simulink model "Modele_LQR_6DOF"  (R2024b)
settings: Solver=VariableStepAuto  StartTime=0.0  StopTime=50  FixedStep=0.0001  RelTol=1e-3
InitFcn:
  |     du0 = 0;
  |     du1 = 0;
  |     du2 = 0;
  |     du3 = 0;
  |     du4 = 0;
  |     du5 = 0;
  |     du6 = 0;
  |     du7 = 0;
values from neighbouring files (symbols this model uses):
  A_num = [0 0 0 0 0 0 0 0 0 0 0 0 ... (144 elements, 12x12)]    [Matrice_A_lineaire.mat]    (also in calcul_matrice_A_lineaire.m = double(A_num); resultats_stabilite.mat; testFinale.m = A_fcn(0, 0, 0, val_rll, val_ptc, val_yw, val_u, val_v, val_w; test_calcalV2.m = double(A_num))
  B = df_dcontrol    [Generate_PyMatrix.m]    (also in Parameters.m = -234.459; instabiliter_graphique.m = out.B_s.signals.values)
  Fx1 = -0.7071*force    (= -14.142)    [Parameters.m]
  Fx2 = -0.7071*force    (= -14.142)    [Parameters.m]
  Fx3 = 0    [Parameters.m]
  Fx4 = 0    [Parameters.m]
  Fx5 = 0    [Parameters.m]
  Fx6 = 0    [Parameters.m]
  Fx7 = 0.7071*force    (= 14.142)    [Parameters.m]
  Fx8 = 0.7071*force    (= 14.142)    [Parameters.m]
  Fy1 = 0.7071*force    (= 14.142)    [Parameters.m]
  Fy2 = -0.7071*force    (= -14.142)    [Parameters.m]
  Fy3 = 0    [Parameters.m]
  Fy4 = 0    [Parameters.m]
  Fy5 = 0    [Parameters.m]
  Fy6 = 0    [Parameters.m]
  Fy7 = 0.7071*force    (= 14.142)    [Parameters.m]
  Fy8 = -0.7071*force    (= -14.142)    [Parameters.m]
  Fz1 = 0    [Parameters.m]
  Fz2 = 0    [Parameters.m]
  Fz3 = -1*force    (= -20)    [Parameters.m]
  Fz4 = -1*force    (= -20)    [Parameters.m]
  Fz5 = -1*force    (= -20)    [Parameters.m]
  Fz6 = -1*force    (= -20)    [Parameters.m]
  Fz7 = 0    [Parameters.m]
  Fz8 = 0    [Parameters.m]
  I_x = 0.578    [Parameters.m]
  I_y = 0.645    [Parameters.m]
  I_z = 0.9366    [Parameters.m]
  lx1 = I_un_moteur(1)    [Calcul_Inertie_Nouveau.m]    (also in Parameters.m = 0.0194)
  lx2 = I_un_moteur(1)    [Calcul_Inertie_Nouveau.m]    (also in Parameters.m = 0.0194)
  lx3 = I_un_moteur(1)    [Calcul_Inertie_Nouveau.m]    (also in Parameters.m = -0.0317)
  lx4 = I_un_moteur(1)    [Calcul_Inertie_Nouveau.m]    (also in Parameters.m = -0.0317)
  lx5 = I_un_moteur(1)    [Calcul_Inertie_Nouveau.m]    (also in Parameters.m = 0.0317)
  lx6 = I_un_moteur(1)    [Calcul_Inertie_Nouveau.m]    (also in Parameters.m = 0.0317)
  lx7 = I_un_moteur(1)    [Calcul_Inertie_Nouveau.m]    (also in Parameters.m = -0.0194)
  lx8 = I_un_moteur(1)    [Calcul_Inertie_Nouveau.m]    (also in Parameters.m = -0.0194)
  ly1 = %.4f    [Calcul_Inertie_Nouveau.m]    (also in Parameters.m = 0.0381)
  ly2 = %.4f    [Calcul_Inertie_Nouveau.m]    (also in Parameters.m = -0.0381)
  ly3 = %.4f    [Calcul_Inertie_Nouveau.m]    (also in Parameters.m = 0.0049)
  ly4 = %.4f    [Calcul_Inertie_Nouveau.m]    (also in Parameters.m = -0.0049)
  ly5 = %.4f    [Calcul_Inertie_Nouveau.m]    (also in Parameters.m = 0.0049)
  ly6 = %.4f    [Calcul_Inertie_Nouveau.m]    (also in Parameters.m = -0.0049)
  ly7 = %.4f    [Calcul_Inertie_Nouveau.m]    (also in Parameters.m = 0.0381)
  ly8 = %.4f    [Calcul_Inertie_Nouveau.m]    (also in Parameters.m = -0.0381)
  lz1 = %.4f;\n', lx1, ly1, lz1)    [Calcul_Inertie_Nouveau.m]    (also in Parameters.m = 0.0575)
  lz2 = %.4f;\n', lx2, ly2, lz2)    [Calcul_Inertie_Nouveau.m]    (also in Parameters.m = 0.0575)
  lz3 = %.4f;\n', lx3, ly3, lz3)    [Calcul_Inertie_Nouveau.m]    (also in Parameters.m = 0.0366)
  lz4 = %.4f;\n', lx4, ly4, lz4)    [Calcul_Inertie_Nouveau.m]    (also in Parameters.m = 0.0366)
  lz5 = %.4f;\n', lx5, ly5, lz5)    [Calcul_Inertie_Nouveau.m]    (also in Parameters.m = 0.0366)
  lz6 = %.4f;\n', lx6, ly6, lz6)    [Calcul_Inertie_Nouveau.m]    (also in Parameters.m = 0.0366)
  lz7 = %.4f;\n', lx7, ly7, lz7)    [Calcul_Inertie_Nouveau.m]    (also in Parameters.m = 0.0575)
  lz8 = %.4f;\n', lx8, ly8, lz8)    [Calcul_Inertie_Nouveau.m]    (also in Parameters.m = 0.0575)
  m = 23.9    [Parameters.m]
  Q_envoyer = Q_final(:,:,1)    [Parameters.m]
  W = mass*gravity    (= 234.459)    [Generate_PyMatrix.m]    (also in Parameters.m; calcul_damping.m)
  x_rb = 0    [Parameters.m]
  x_rg = 0    [Parameters.m]
  y_rb = 0    [Parameters.m]
  y_rg = 0    [Parameters.m]
  z_rb = 0    [Parameters.m]
  z_rg = 0    [Parameters.m]
undefined symbols (not defined in the file or in its folder): sigbuilder_block
libraries: simulink x12, sharedtransform x1, dspinverses x1, SignalEditorBlockLib x1
(part 2 of 4)

== matlab function Modele_LQR_6DOF/ROV model/ROV model/Kinetics1 ==
  data: u input size=1; u_dot output; v input size=1; w input size=1; p input size=1; q input size=1; r input size=1; phi input; theta input; psi input; tau input; v_dot output; w_dot output; p_dot output; q_dot output; r_dot output; u_dot_temp input; v_dot_temp input; w_dot_temp input; p_dot_temp input; q_dot_temp input; r_dot_temp input; disturbance input; EstimatedParams input; B parameter; Fx1 input; Fx2 input; Fx3 input; Fx4 input; Fx5 input; Fx6 input; Fx7 input; Fx8 input; Fy1 input; Fy2 input; Fy3 input; Fy4 input; Fy5 input; Fy6 input; Fy7 input; Fy8 input; Fz1 input; Fz2 input; Fz3 input; Fz4 input; Fz5 input; Fz6 input; Fz7 input; Fz8 input; I_x input; I_y input; I_z input; lx1 input; lx2 input; lx3 input; lx4 input; lx5 input; lx6 input; lx7 input; lx8 input; ly1 input; ly2 input; ly3 input; ly4 input; ly5 input; ly6 input; ly7 input; ly8 input; lz1 input; lz2 input; lz3 input; lz4 input; lz5 input; lz6 input; lz7 input; lz8 input; m parameter; W parameter; x_rb parameter; x_rg parameter; y_rb parameter; y_rg parameter; z_rb parameter; z_rg parameter
function [u_dot,v_dot,w_dot,p_dot,q_dot,r_dot] = Kinetics1(u,v,w,p,q,r,phi,theta,psi,tau,u_dot_temp,v_dot_temp,w_dot_temp,p_dot_temp,q_dot_temp,r_dot_temp, disturbance,EstimatedParams, B, Fx1, Fx2, Fx3, Fx4, Fx5, Fx6, Fx7, Fx8, Fy1, Fy2, Fy3, Fy4, Fy5, Fy6, Fy7, Fy8, Fz1, Fz2, Fz3, Fz4, Fz5, Fz6, Fz7, Fz8, I_x, I_y, I_z, lx1, lx2, lx3, lx4, lx5, lx6, lx7, lx8, ly1, ly2, ly3, ly4, ly5, ly6, ly7, ly8, lz1, lz2, lz3, lz4, lz5, lz6, lz7, lz8, m, W, x_rb, x_rg, y_rb, y_rg, z_rb, z_rg)
% LIVRE HMCH PAGE 58
%extract forces from thrusters
f1=tau(1);
f2=tau(2);
f3=tau(3);
f4=tau(4);
f5=tau(5);
f6=tau(6);
f7=tau(7);
f8=tau(8);
x_rb = 0; x_rg = 0; y_rb = 0; y_rg = 0; z_rb = -0.05; z_rg = 0;
  displaced_water_volume = 0.024; % 0.03
  water_density = 1000.0;
  radius = 0.26;
  m = 23.9;
  g = 9.81;
  W = m * g;
  B = water_density*displaced_water_volume*g;
  % B = W;
%extract estimated parameters
X_u = EstimatedParams(1);
Y_v = EstimatedParams(2);
Z_w = EstimatedParams(3);
K_p = EstimatedParams(4); 
M_q = EstimatedParams(5);
N_r = EstimatedParams(6);
X_uu = EstimatedParams(7);
Y_vv = EstimatedParams(8);
Z_ww = EstimatedParams(9);
K_pp = EstimatedParams(10); 
M_qq = EstimatedParams(11); 
N_rr = EstimatedParams(12);
X_u_dot = EstimatedParams(13);
Y_v_dot = EstimatedParams(14);
Z_w_dot = EstimatedParams(15);
K_p_dot = EstimatedParams(16);
M_q_dot = EstimatedParams(17); 
N_r_dot = EstimatedParams(18); 
%extract forces from disturbance
u_c = disturbance(1);
v_c = disturbance(2);
w_c = disturbance(3);
p_c = disturbance(4);
q_c = disturbance(5);
r_c = disturbance(6);
%Full Equations without disturbance with zg = 0.02
% u_dot = -((0.7071*f1) + (0.7071*f2) - (0.7071*f3) - (0.7071*f4)- (0.230*q_dot_temp) + 2*sin(theta) + u*(X_u + X_uu*abs(u)) - (0.230*p*r) - (11.50*q*w) + (11.50*r*v) - Y_v_dot*r*v + Z_w_dot*q*w)/(X_u_dot - 11.50);
% v_dot = ((0.7071*f1) - (0.7071*f2) + (0.7071*f3) - (0.7071*f4) - (0.230*p_dot_temp) + 2*cos(theta)*sin(phi) - v*(Y_v + Y_vv*abs(v)) + (11.50*q*r) - (11.50*p*w) + (11.50*r*u) - X_u_dot*r*u + Z_w_dot*p*w)/(Y_v_dot - 11.50);
% w_dot = -(f6 - f5 + f7 - f8 - 2*cos(phi)*cos(theta) + w*(Z_w + Z_ww*abs(w)) + q*((23*q)/100 - X_u_dot*u) + p*((23*p)/100 + Y_v_dot*v) - (11.50*p*v) + (11.50*q*u))/(Z_w_dot - 11.50);
% p_dot = -(25*((0.0601*f1) - (0.0601*f2) + (0.0601*f3) - (0.0601*f4) - (109*f5)/500 - (109*f6)/500 + (0.2180*f7) + (0.2180*f8) + (0.230*v_dot_temp) + K_p*p - (2.2560*cos(theta)*sin(phi)) - (0.230*p*w) + (0.230*r*u) - M_q_dot*q*r + N_r_dot*q*r - Y_v_dot*v*w + Z_w_dot*v*w + K_pp*p*abs(p)))/(25*K_p_dot - 4);
% q_dot =-(25*((0.0601*f1) + (0.0601*f2) - (0.0601*f3) - (0.0601*f4)+ (0.120*f5) - (0.120*f6) + (0.120*f7) - (0.120*f8) - (0.230*u_dot_temp) - (2.2560*sin(theta)) + M_q*q - (0.230*q*w) + (0.230*r*v) + K_p_dot*p*r - N_r_dot*p*r + X_u_dot*u*w - Z_w_dot*u*w + M_qq*q*abs(q)))/(25*M_q_dot - 4);
% r_dot = -(25*((0.1888*f2) - (0.1888*f1) + (0.1888*f3) - (0.1888*f4) + N_r*r - K_p_dot*p*q + M_q_dot*p*q - X_u_dot*u*v + Y_v_dot*u*v + N_rr*r*abs(r)))/(25*N_r_dot - 4);

%Full Equations without disturbance with zg = 0.02 + utilisation de la fontion vpa
% u_dot = -(1.0*(0.7071*f1 + 0.7071*f2 - 0.7071*f3 - 0.7071*f4 - 0.23*q_dot_temp + 2.0*sin(theta) + (X_u + X_uu*abs(u - 1.0*u_c))*(u - 1.0*u_c) - 1.0*(11.5*q - 11.5*q_c)*(w - 1.0*w_c) + (11.5*r - 11.5*r_c)*(v - 1.0*v_c) - 1.0*(p - 1.0*p_c)*(0.23*r - 0.23*r_c) + (X_u_dot - 11.5)*(q*w_c - 1.0*r*v_c) - 1.0*Y_v_dot*(r - 1.0*r_c)*(v - 1.0*v_c) + Z_w_dot*(q - 1.0*q_c)*(w - 1.0*w_c)))/(X_u_dot - 11.5);
% v_dot = (0.7071*f1 - 0.7071*f2 + 0.7071*f3 - 0.7071*f4 - 0.23*p_dot_temp - 1.0*(11.5*p - 11.5*p_c)*(w - 1.0*w_c) + (11.5*r - 11.5*r_c)*(u - 1.0*u_c) - 1.0*(Y_v + Y_vv*abs(v - 1.0*v_c))*(v - 1.0*v_c) + 2.0*cos(theta)*sin(phi) + (q - 1.0*q_c)*(0.23*r - 0.23*r_c) + (Y_v_dot - 11.5)*(p*w_c - 1.0*r*u_c) - 1.0*X_u_dot*(r - 1.0*r_c)*(u - 1.0*u_c) + Z_w_dot*(p - 1.0*p_c)*(w - 1.0*w_c))/(Y_v_dot - 11.5);
% w_dot =-(1.0*(f6 - 1.0*f5 + f7 - 1.0*f8 - 1.0*(11.5*p - 11.5*p_c)*(v - 1.0*v_c) + (11.5*q - 11.5*q_c)*(u - 1.0*u_c) - 2.0*cos(phi)*cos(theta) + (Z_w + Z_ww*abs(w - 1.0*w_c))*(w - 1.0*w_c) + (Z_w_dot - 11.5)*(p*v_c - 1.0*q*u_c) + (p - 1.0*p_c)*(0.23*p - 0.23*p_c + Y_v_dot*(v - 1.0*v_c)) - 1.0*(q - 1.0*q_c)*(0.23*q_c - 0.23*q + X_u_dot*(u - 1.0*u_c))))/(Z_w_dot - 11.5);
% p_dot =-(1.0*(0.0601035*f1 - 0.0601035*f2 + 0.0601035*f3 - 0.0601035*f4 - 0.218*f5 - 0.218*f6 + 0.218*f7 + 0.218*f8 + 0.23*v_dot - 2.256*cos(theta)*sin(phi) + (u - 1.0*u_c)*(0.23*r - 0.23*r_c) - 0.23*p*w_c + 0.23*r*u_c - 1.0*(r - 1.0*r_c)*(0.16*q_c - 0.16*q + M_q_dot*(q - 1.0*q_c)) + (q - 1.0*q_c)*(0.16*r_c - 0.16*r + N_r_dot*(r - 1.0*r_c)) + (K_p + K_pp*abs(p - 1.0*p_c))*(p - 1.0*p_c) - 1.0*(w - 1.0*w_c)*(0.23*p - 0.23*p_c + Y_v_dot*(v - 1.0*v_c)) + Z_w_dot*(v - 1.0*v_c)*(w - 1.0*w_c)))/(K_p_dot - 0.16);
% q_dot =-(1.0*(0.0601035*f1 + 0.0601035*f2 - 0.0601035*f3 - 0.0601035*f4 + 0.12*f5 - 0.12*f6 + 0.12*f7 - 0.12*f8 - 0.23*u_dot - 2.256*sin(theta) + (v - 1.0*v_c)*(0.23*r - 0.23*r_c) - 0.23*q*w_c + 0.23*r*v_c + (r - 1.0*r_c)*(0.16*p_c - 0.16*p + K_p_dot*(p - 1.0*p_c)) - 1.0*(p - 1.0*p_c)*(0.16*r_c - 0.16*r + N_r_dot*(r - 1.0*r_c)) + (w - 1.0*w_c)*(0.23*q_c - 0.23*q + X_u_dot*(u - 1.0*u_c)) + (M_q + M_qq*abs(q - 1.0*q_c))*(q - 1.0*q_c) - 1.0*Z_w_dot*(u - 1.0*u_c)*(w - 1.0*w_c)))/(M_q_dot - 0.16);
% r_dot = -(1.0*(0.1887957*f2 - 0.1887957*f1 + 0.1887957*f3 - 0.1887957*f4 - 1.0*(q - 1.0*q_c)*(0.16*p_c - 0.16*p + K_p_dot*(p - 1.0*p_c)) + (p - 1.0*p_c)*(0.16*q_c - 0.16*q + M_q_dot*(q - 1.0*q_c)) + (N_r + N_rr*abs(r - 1.0*r_c))*(r - 1.0*r_c) - 1.0*X_u_dot*(u - 1.0*u_c)*(v - 1.0*v_c) + Y_v_dot*(u - 1.0*u_c)*(v - 1.0*v_c)))/(N_r_dot - 0.16);

% u_dot = -(1.0*((X_u + X_uu*abs(u - 1.0*u_c))*(u - 1.0*u_c) + sin(theta)*(B - 9.81*m) + Fx1*f1 + Fx2*f2 + Fx3*f3 + Fx4*f4 + Fx5*f5 + Fx6*f6 + Fx7*f7 + Fx8*f8 + (q*w_c - 1.0*r*v_c)*(X_u_dot - 1.0*m) + (Z_w_dot*(w - 1.0*w_c) + m*x_rg*(q - 1.0*q_c))*(q - 1.0*q_c) - 1.0*(Y_v_dot*(v - 1.0*v_c) - 1.0*m*x_rg*(r - 1.0*r_c))*(r - 1.0*r_c) - 1.0*(m*y_rg*(q - 1.0*q_c) + m*z_rg*(r - 1.0*r_c))*(p - 1.0*p_c) - 1.0*m*(q - 1.0*q_c)*(w - 1.0*w_c) + m*(r - 1.0*r_c)*(v - 1.0*v_c) - 1.0*m*q_dot_temp*z_rg + m*r_dot_temp*y_rg))/(X_u_dot - 1.0*m);
%  
%  
% v_dot = -(1.0*((Y_v + Y_vv*abs(v - 1.0*v_c))*(v - 1.0*v_c) + Fy1*f1 + Fy2*f2 + Fy3*f3 + Fy4*f4 + Fy5*f5 + Fy6*f6 + Fy7*f7 + Fy8*f8 - 1.0*(p*w_c - 1.0*r*u_c)*(Y_v_dot - 1.0*m) + (X_u_dot*(u - 1.0*u_c) + m*y_rg*(r - 1.0*r_c))*(r - 1.0*r_c) - 1.0*(Z_w_dot*(w - 1.0*w_c) - 1.0*m*y_rg*(p - 1.0*p_c))*(p - 1.0*p_c) - 1.0*(m*x_rg*(p - 1.0*p_c) + m*z_rg*(r - 1.0*r_c))*(q - 1.0*q_c) + m*(p - 1.0*p_c)*(w - 1.0*w_c) - 1.0*m*(r - 1.0*r_c)*(u - 1.0*u_c) + m*p_dot_temp*z_rg - 1.0*m*r_dot_temp*x_rg - 1.0*cos(theta)*sin(phi)*(B - 9.81*m)))/(Y_v_dot - 1.0*m);
%  
%  
% w_dot = -(1.0*(Fz1*f1 + Fz2*f2 + Fz3*f3 + Fz4*f4 + Fz5*f5 + Fz6*f6 + Fz7*f7 + Fz8*f8 + (Z_w + Z_ww*abs(w - 1.0*w_c))*(w - 1.0*w_c) + (p*v_c - 1.0*q*u_c)*(Z_w_dot - 1.0*m) + (Y_v_dot*(v - 1.0*v_c) + m*z_rg*(p - 1.0*p_c))*(p - 1.0*p_c) - 1.0*(X_u_dot*(u - 1.0*u_c) - 1.0*m*z_rg*(q - 1.0*q_c))*(q - 1.0*q_c) - 1.0*(m*x_rg*(p - 1.0*p_c) + m*y_rg*(q - 1.0*q_c))*(r - 1.0*r_c) - 1.0*m*(p - 1.0*p_c)*(v - 1.0*v_c) + m*(q - 1.0*q_c)*(u - 1.0*u_c) - 1.0*m*p_dot_temp*y_rg + m*q_dot_temp*x_rg - 1.0*cos(phi)*cos(theta)*(B - 9.81*m)))/(Z_w_dot - 1.0*m);
%  
%  
% p_dot = -(1.0*((Y_v_dot*(v - 1.0*v_c) + m*z_rg*(p - 1.0*p_c))*(w - 1.0*w_c) + f1*(Fy1*lz1 - 1.0*Fz1*ly1) + f2*(Fy2*lz2 - 1.0*Fz2*ly2) + f3*(Fy3*lz3 - 1.0*Fz3*ly3) + f4*(Fy4*lz4 - 1.0*Fz4*ly4) + f5*(Fy5*lz5 - 1.0*Fz5*ly5) + f6*(Fy6*lz6 - 1.0*Fz6*ly6) + f7*(Fy7*lz7 - 1.0*Fz7*ly7) + f8*(Fy8*lz8 - 1.0*Fz8*ly8) - 1.0*(Z_w_dot*(w - 1.0*w_c) - 1.0*m*y_rg*(p - 1.0*p_c))*(v - 1.0*v_c) - 1.0*(K_p + K_pp*abs(p - 1.0*p_c))*(p - 1.0*p_c) - 1.0*(m*y_rg*(q - 1.0*q_c) + m*z_rg*(r - 1.0*r_c))*(u - 1.0*u_c) - 1.0*(I_y*(q - 1.0*q_c) - 1.0*M_q_dot*(q - 1.0*q_c))*(r - 1.0*r_c) + (I_z*(r - 1.0*r_c) - 1.0*N_r_dot*(r - 1.0*r_c))*(q - 1.0*q_c) + cos(phi)*cos(theta)*(B*y_rb - 9.81*m*y_rg) - 1.0*cos(theta)*sin(phi)*(B*z_rb - 9.81*m*z_rg) + m*y_rg*(w_dot + p*v_c - 1.0*q*u_c) - 1.0*m*z_rg*(v_dot - 1.0*p*w_c + r*u_c)))/(I_x - 1.0*K_p_dot);
%  
%  
% q_dot = (sin(theta)*(B*z_rb - 9.81*m*z_rg) - 1.0*(Z_w_dot*(w - 1.0*w_c) + m*x_rg*(q - 1.0*q_c))*(u - 1.0*u_c) + f1*(Fx1*lz1 - 1.0*Fz1*lx1) + f2*(Fx2*lz2 - 1.0*Fz2*lx2) + f3*(Fx3*lz3 - 1.0*Fz3*lx3) + f4*(Fx4*lz4 - 1.0*Fz4*lx4) + f5*(Fx5*lz5 - 1.0*Fz5*lx5) + f6*(Fx6*lz6 - 1.0*Fz6*lx6) + f7*(Fx7*lz7 - 1.0*Fz7*lx7) + f8*(Fx8*lz8 - 1.0*Fz8*lx8) + (X_u_dot*(u - 1.0*u_c) - 1.0*m*z_rg*(q - 1.0*q_c))*(w - 1.0*w_c) + (M_q + M_qq*abs(q - 1.0*q_c))*(q - 1.0*q_c) - 1.0*(I_x*(p - 1.0*p_c) - 1.0*K_p_dot*(p - 1.0*p_c))*(r - 1.0*r_c) + (m*x_rg*(p - 1.0*p_c) + m*z_rg*(r - 1.0*r_c))*(v - 1.0*v_c) + (I_z*(r - 1.0*r_c) - 1.0*N_r_dot*(r - 1.0*r_c))*(p - 1.0*p_c) + cos(phi)*cos(theta)*(B*x_rb - 9.81*m*x_rg) + m*x_rg*(w_dot + p*v_c - 1.0*q*u_c) - 1.0*m*z_rg*(u_dot + q*w_c - 1.0*r*v_c))/(I_y - 1.0*M_q_dot);
%  
%  
% r_dot = -(1.0*(sin(theta)*(B*y_rb - 9.81*m*y_rg) + (X_u_dot*(u - 1.0*u_c) + m*y_rg*(r - 1.0*r_c))*(v - 1.0*v_c) + f1*(Fx1*ly1 - 1.0*Fy1*lx1) + f2*(Fx2*ly2 - 1.0*Fy2*lx2) + f3*(Fx3*ly3 - 1.0*Fy3*lx3) + f4*(Fx4*ly4 - 1.0*Fy4*lx4) + f5*(Fx5*ly5 - 1.0*Fy5*lx5) + f6*(Fx6*ly6 - 1.0*Fy6*lx6) + f7*(Fx7*ly7 - 1.0*Fy7*lx7) + f8*(Fx8*ly8 - 1.0*Fy8*lx8) - 1.0*(Y_v_dot*(v - 1.0*v_c) - 1.0*m*x_rg*(r - 1.0*r_c))*(u - 1.0*u_c) - 1.0*(N_r + N_rr*abs(r - 1.0*r_c))*(r - 1.0*r_c) - 1.0*(I_x*(p - 1.0*p_c) - 1.0*K_p_dot*(p - 1.0*p_c))*(q - 1.0*q_c) + (I_y*(q - 1.0*q_c) - 1.0*M_q_dot*(q - 1.0*q_c))*(p - 1.0*p_c) - 1.0*(m*x_rg*(p - 1.0*p_c) + m*y_rg*(q - 1.0*q_c))*(w - 1.0*w_c) + cos(theta)*sin(phi)*(B*x_rb - 9.81*m*x_rg) + m*x_rg*(v_dot - 1.0*p*w_c + r*u_c) - 1.0*m*y_rg*(u_dot + q*w_c - 1.0*r*v_c)))/(I_z - 1.0*N_r_dot);
%--------------------------------------------------------------------------%
u_dot = -(1.0 * ( ...
    (X_u + X_uu*abs(u - 1.0*u_c))*(u - 1.0*u_c) ...
    + Fx1*f1 + Fx2*f2 + Fx3*f3 + Fx4*f4 ...
    + Fx5*f5 + Fx6*f6 + Fx7*f7 + Fx8*f8 ...
    + (q*w_c - 1.0*r*v_c)*(X_u_dot - 1.0*m) ...
    + (Z_w_dot*(w - 1.0*w_c) + m*x_rg*(q - 1.0*q_c))*(q - 1.0*q_c) ...
    - 1.0*(Y_v_dot*(v - 1.0*v_c) - 1.0*m*x_rg*(r - 1.0*r_c))*(r - 1.0*r_c) ...
    + sin(theta)*(W - 1.0*B) ...
    - 1.0*(m*y_rg*(q - 1.0*q_c) + m*z_rg*(r - 1.0*r_c))*(p - 1.0*p_c) ...
    - 1.0*m*(q - 1.0*q_c)*(w - 1.0*w_c) ...
    + m*(r - 1.0*r_c)*(v - 1.0*v_c) ...
    - 1.0*m*q_dot_temp*z_rg ...
    + m*r_dot_temp*y_rg ...
    )) / (X_u_dot - 1.0*m);

%--------------------------------------------------------------------------%
v_dot = -(1.0 * ( ...
    (Y_v + Y_vv*abs(v - 1.0*v_c))*(v - 1.0*v_c) ...
    + Fy1*f1 + Fy2*f2 + Fy3*f3 + Fy4*f4 ...
    + Fy5*f5 + Fy6*f6 + Fy7*f7 + Fy8*f8 ...
    - 1.0*(p*w_c - 1.0*r*u_c)*(Y_v_dot - 1.0*m) ...
    + (X_u_dot*(u - 1.0*u_c) + m*y_rg*(r - 1.0*r_c))*(r - 1.0*r_c) ...
    - 1.0*(Z_w_dot*(w - 1.0*w_c) - 1.0*m*y_rg*(p - 1.0*p_c))*(p - 1.0*p_c) ...
    - 1.0*(m*x_rg*(p - 1.0*p_c) + m*z_rg*(r - 1.0*r_c))*(q - 1.0*q_c) ...
    + m*(p - 1.0*p_c)*(w - 1.0*w_c) ...
    - 1.0*m*(r - 1.0*r_c)*(u - 1.0*u_c) ...
    - 1.0*cos(theta)*sin(phi)*(W - 1.0*B) ...
    + m*p_dot_temp*z_rg ...
    - 1.0*m*r_dot_temp*x_rg ...
    )) / (Y_v_dot - 1.0*m);
%--------------------------------------------------------------------------%
w_dot = -(1.0 * ( ...
    Fz1*f1 + Fz2*f2 + Fz3*f3 + Fz4*f4 ...
    + Fz5*f5 + Fz6*f6 + Fz7*f7 + Fz8*f8 ...
    + (Z_w + Z_ww*abs(w - 1.0*w_c))*(w - 1.0*w_c) ...
    + (p*v_c - 1.0*q*u_c)*(Z_w_dot - 1.0*m) ...
    + (Y_v_dot*(v - 1.0*v_c) + m*z_rg*(p - 1.0*p_c))*(p - 1.0*p_c) ...
    - 1.0*(X_u_dot*(u - 1.0*u_c) - 1.0*m*z_rg*(q - 1.0*q_c))*(q - 1.0*q_c) ...
    - 1.0*(m*x_rg*(p - 1.0*p_c) + m*y_rg*(q - 1.0*q_c))*(r - 1.0*r_c) ...
    - 1.0*m*(p - 1.0*p_c)*(v - 1.0*v_c) ...
    + m*(q - 1.0*q_c)*(u - 1.0*u_c) ...
    - 1.0*cos(phi)*cos(theta)*(W - 1.0*B) ...
    - 1.0*m*p_dot_temp*y_rg ...
    + m*q_dot_temp*x_rg ...
    )) / (Z_w_dot - 1.0*m);

%--------------------------------------------------------------------------%
p_dot = -(1.0 * ( ...
    (Y_v_dot*(v - 1.0*v_c) + m*z_rg*(p - 1.0*p_c))*(w - 1.0*w_c) ...
    - 1.0*cos(theta)*( ...
        W*y_rg*cos(phi) ...
        - 1.0*W*z_rg*sin(phi) ...
        - 1.0*B*y_rb*cos(phi) ...
        + B*z_rb*sin(phi)) ...
    + f1*(Fy1*lz1 - 1.0*Fz1*ly1) ...
    + f2*(Fy2*lz2 - 1.0*Fz2*ly2) ...
    + f3*(Fy3*lz3 - 1.0*Fz3*ly3) ...
    + f4*(Fy4*lz4 - 1.0*Fz4*ly4) ...
    + f5*(Fy5*lz5 - 1.0*Fz5*ly5) ...
    + f6*(Fy6*lz6 - 1.0*Fz6*ly6) ...
    + f7*(Fy7*lz7 - 1.0*Fz7*ly7) ...
    + f8*(Fy8*lz8 - 1.0*Fz8*ly8) ...
    - 1.0*(Z_w_dot*(w - 1.0*w_c) - 1.0*m*y_rg*(p - 1.0*p_c))*(v - 1.0*v_c) ...
    - 1.0*(K_p + K_pp*abs(p - 1.0*p_c))*(p - 1.0*p_c) ...
    - 1.0*(m*y_rg*(q - 1.0*q_c) + m*z_rg*(r - 1.0*r_c))*(u - 1.0*u_c) ...
    - 1.0*(I_y*(q - 1.0*q_c) - 1.0*M_q_dot*(q - 1.0*q_c))*(r - 1.0*r_c) ...
    + (I_z*(r - 1.0*r_c) - 1.0*N_r_dot*(r - 1.0*r_c))*(q - 1.0*q_c) ...
    + m*y_rg*(w_dot + p*v_c - 1.0*q*u_c) ...
    - 1.0*m*z_rg*(v_dot - 1.0*p*w_c + r*u_c) ...
    )) / (I_x - 1.0*K_p_dot);

%--------------------------------------------------------------------------%
q_dot = ( ...
    f1*(Fx1*lz1 - 1.0*Fz1*lx1) ...
    - 1.0*(Z_w_dot*(w - 1.0*w_c) + m*x_rg*(q - 1.0*q_c))*(u - 1.0*u_c) ...
    + f2*(Fx2*lz2 - 1.0*Fz2*lx2) ...
    + f3*(Fx3*lz3 - 1.0*Fz3*lx3) ...
    + f4*(Fx4*lz4 - 1.0*Fz4*lx4) ...
    + f5*(Fx5*lz5 - 1.0*Fz5*lx5) ...
    + f6*(Fx6*lz6 - 1.0*Fz6*lx6) ...
    + f7*(Fx7*lz7 - 1.0*Fz7*lx7) ...
    + f8*(Fx8*lz8 - 1.0*Fz8*lx8) ...
    + (X_u_dot*(u - 1.0*u_c) - 1.0*m*z_rg*(q - 1.0*q_c))*(w - 1.0*w_c) ...
    + (M_q + M_qq*abs(q - 1.0*q_c))*(q - 1.0*q_c) ...
    - 1.0*(I_x*(p - 1.0*p_c) - 1.0*K_p_dot*(p - 1.0*p_c))*(r - 1.0*r_c) ...
    + (m*x_rg*(p - 1.0*p_c) + m*z_rg*(r - 1.0*r_c))*(v - 1.0*v_c) ...
    + (I_z*(r - 1.0*r_c) - 1.0*N_r_dot*(r - 1.0*r_c))*(p - 1.0*p_c) ...
    + B*z_rb*sin(theta) ...
    - 1.0*W*z_rg*sin(theta) ...
    + m*x_rg*(w_dot + p*v_c - 1.0*q*u_c) ...
    - 1.0*m*z_rg*(u_dot + q*w_c - 1.0*r*v_c) ...
    + B*x_rb*cos(phi)*cos(theta) ...
    - 1.0*W*x_rg*cos(phi)*cos(theta) ...
    ) / (I_y - 1.0*M_q_dot);

%--------------------------------------------------------------------------%
r_dot = -(1.0 * ( ...
    (X_u_dot*(u - 1.0*u_c) + m*y_rg*(r - 1.0*r_c))*(v - 1.0*v_c) ...
    + f1*(Fx1*ly1 - 1.0*Fy1*lx1) ...
    + f2*(Fx2*ly2 - 1.0*Fy2*lx2) ...
    + f3*(Fx3*ly3 - 1.0*Fy3*lx3) ...
    + f4*(Fx4*ly4 - 1.0*Fy4*lx4) ...
    + f5*(Fx5*ly5 - 1.0*Fy5*lx5) ...
    + f6*(Fx6*ly6 - 1.0*Fy6*lx6) ...
    + f7*(Fx7*ly7 - 1.0*Fy7*lx7) ...
    + f8*(Fx8*ly8 - 1.0*Fy8*lx8) ...
    - 1.0*(Y_v_dot*(v - 1.0*v_c) - 1.0*m*x_rg*(r - 1.0*r_c))*(u - 1.0*u_c) ...
    - 1.0*(N_r + N_rr*abs(r - 1.0*r_c))*(r - 1.0*r_c) ...
    - 1.0*(I_x*(p - 1.0*p_c) - 1.0*K_p_dot*(p - 1.0*p_c))*(q - 1.0*q_c) ...
    + (I_y*(q - 1.0*q_c) - 1.0*M_q_dot*(q - 1.0*q_c))*(p - 1.0*p_c) ...
    - 1.0*(m*x_rg*(p - 1.0*p_c) + m*y_rg*(q - 1.0*q_c))*(w - 1.0*w_c) ...
    + B*y_rb*sin(theta) ...
    - 1.0*W*y_rg*sin(theta) ...
    + m*x_rg*(v_dot - 1.0*p*w_c + r*u_c) ...
    - 1.0*m*y_rg*(u_dot + q*w_c - 1.0*r*v_c) ...
    + B*x_rb*cos(theta)*sin(phi) ...
    - 1.0*W*x_rg*cos(theta)*sin(phi) ...
    )) / (I_z - 1.0*N_r_dot);

%--------------------------------------------------------------------------%
end
